simulink model "Reference_model_Control_Engineering_2022"  (R2022b)
settings: Solver=FixedStepDiscrete  StartTime=0.0  StopTime=inf  FixedStep=Ts  RelTol=1e-3  EnableMultiTasking=on
InitFcn:
  | Fs = 4000; Ts = 1/Fs; tsim = 29.9997;
settings Model: SimulationMode=external  ExtModeTrigDuration=2  Creator=Enzo  LastModifiedBy=vaish
settings SolverCC: AlgebraicLoopSolver=TrustRegion  PositivePriorityOrder=on
settings DataIOCC: SaveOutput=off  DSMLogging=off  SaveTime=off  ReturnWorkspaceOutputs=off
settings OptimizationCC: ReuseModelBlockBuffer=on  EnhancedBackFolding=on  PassReuseOutputArgsThreshold=0  MaxStackSize=64  OptimizeBlockOrder=speed  DifferentSizesBufferReuse=on  OptimizationCustomize=off
settings DebuggingCC: ParameterTunabilityLossMsg=error  UnconnectedInputMsg=warning  UnconnectedOutputMsg=warning  UnconnectedLineMsg=warning  ArithmeticOperatorsInVariantConditions=warning
settings HardwareCC: ProdBitPerPointer=32  ProdBitPerSizeT=32  ProdBitPerPtrDiffT=32  ProdLargestAtomicInteger=Long  ProdLargestAtomicFloat=Double  ProdWordSize=32  ProdLongLongMode=on  ProdHWDeviceType=ARM Compatible->ARM Cortex  UseEmbeddedCoderFeatures=off
settings ModelReferenceCC: EnableRefExpFcnMdlSchedulingChecks=on
settings SFSimCC: CustomCodeUndefinedFunction=UseInterfaceOnly
settings RTWCC: Description=Embedded Coder  SystemTargetFile=ert.tlc  HardwareBoard=Raspberry Pi  TLCOptions="-aInlineSetEventsForThisBaseRateFcn=TLC_FALSE -aSuppressMultiTaskScheduler=TLC_FALSE  -aRateBasedStepFcn=0"  TemplateMakefile=ert_default_tmf  PostCodeGenCommand="if (~verLessThan('matlab', '9.11')) codertarget.postCodeGenHookCommand(h);  SPERTE_postGenFunc(modelName, buildInfo); else; SPERTE_postGenFunc(h, buildInfo); end"  Toolchain=GNU GCC Embedded Linux  BuildConfiguration=Faster Runs
settings CodeAppCC: ForceParamTrailComments=on  OperatorAnnotations=on
settings ERTTargetCC: ERTCustomFileBanners=off  SupportContinuousTime=on  SupportNonInlinedSFcns=on  RemoveResetFunc=off  SupportVariableSizeSignals=on  ModelStepFunctionPrototypeControlCompliant=off  ExtMode=on  ExtModeMexArgs='sperte0.bwk.tue.nl' 0 17725  ERTSrcFileBannerTemplate=codertarget_code_template.cgt  ERTHdrFileBannerTemplate=codertarget_code_template.cgt  ERTDataSrcFileTemplate=codertarget_code_template.cgt  ERTDataHdrFileTemplate=codertarget_code_template.cgt
settings SettingsController: UseSoCProfilerForTargets=0

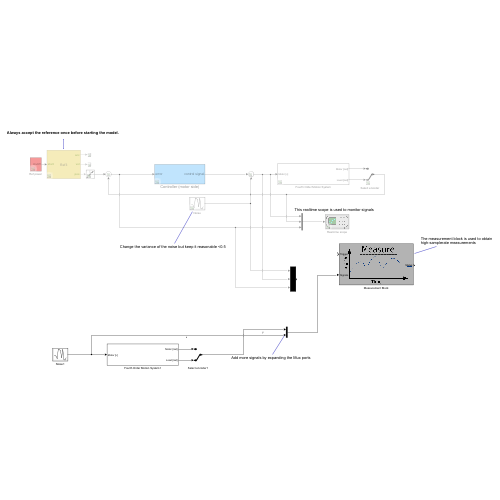
[thumbnail: Simulink's stored preview of the top-level diagram]
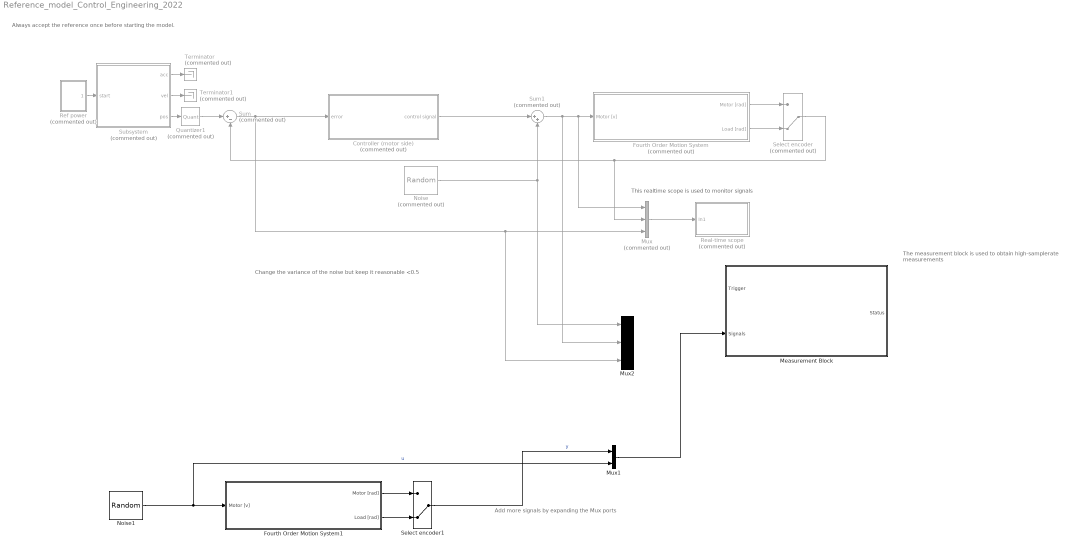
== system Reference_model_Control_Engineering_2022 ==
  note: Add more signals by expanding the Mux ports
  note: The measurement block is used to obtain high-samplerate measurements
  note: This realtime scope is used to monitor signals
  note: Always accept the reference once before starting the model.
  note: Change the variance of the noise but keep it reasonable <0.5
  Controller (motor side) : Subsystem  Commented=on
  Fourth Order Motion System : Subsystem  Commented=on
  Fourth Order Motion System1 : Subsystem
  Measurement Block : Subsystem  Description=|  Priority=-1  mask(SPERTE Lib){N_samples=480000, triggertype=2, trigger_command=0}
      | Perform on-demand measurements to file using this block.
      | 
      | It can be used in 2 ways:
      | 1) Set the mask triggertype parameter to manual and use the trigger input signal to trigger a measurement.
      | You can do this by providing a 0 to 1 transition.
      | Keep it low after you start/complete the measurement, or it will measure again.
      | A file is created with measurement_0,1,2... etc
      | 
      | 2) Keep the model running, and trigger a measurement from the commandline or Matlab script.
      | For example:
      | 
      | % How many samples to measure?
      | N_samples = Fs*5;
      | % Do the measurement
      | SPERTE_Perform_Measurement(N_samples);
      | % Get the latest file
      | file_list = SPERTE_Get_Latest_Measurement(p,1,'./data');
      | % How many signals did you record?
      | N_signals = 3;
      | % Convert the .bin to .mat and return the results
      | measurement = SPERTE_Bin_To_Mat(file_list,N_signals);
      mask prompts: N_samples "Number of samples"; trigger_command "Trigger command"
      mask help:
      | This block implements a measurement to file sink.
      | It can be used in two ways:
      | 1) Triggered from the simulink model
      | 2) Triggered from the command line
      mask Help:
      | Perform on-demand measurements to file using this block.
      | 
      | It can be used in 2 ways:
      | 1) Set the mask triggertype parameter to manual and use the trigger input signal to trigger a measurement.
      | You can do this by providing a 0 to 1 transition.
      | Keep it low after you start/complete the measurement, or it will measure again.
      | A file is created with measurement_0,1,2... etc
      | 
      | 2) Keep the model running, and trigger a measurement from the commandline or Matlab script.
      | For example:
      | 
      | % How many samples to measure?
      | N_samples = Fs*5;
      | % Do the measurement
      | SPERTE_Perform_Measurement(N_samples);
      | % Get the latest file
      | file_list = SPERTE_Get_Latest_Measurement(p,1,'./data');
      | % How many signals did you record?
      | N_signals = 3;
      | % Convert the .bin to .mat and return the results
      | measurement = SPERTE_Bin_To_Mat(file_list,N_signals);
      mask TypeOptions N_samples: SPERTE_measurement_samples/Value
      mask TypeOptions trigger_command: SPERTE_measurement_trigger_command/Value
      mask DialogControl BlockName Prompt: Sperte measurement block.
      mask DialogControl Desc Prompt: Can be used to trace signals to .bin file on the Raspberry Pi.  Can be triggered through signals in the simulink model or manually.
      mask DialogControl TriggerText Prompt: Manual (0), Command (1), Both (2)
      mask Display: ud = get_param(gcb,'UserData');image(ud.x);
  Mux : Mux  Commented=on  Inputs=3
  Mux1 : Mux  Inputs=2
  Mux2 : Mux  Inputs=3
  Noise : RandomNumber  Commented=on  SampleTime=Ts
  Noise1 : RandomNumber  SampleTime=Ts
  Quantizer1 : Quantizer  Commented=on  QuantizationInterval=(2*pi)/(500*4)
  Real-time scope : Subsystem  Priority=0  Commented=on  mask(Scope){Sample_Time=1/500}
      mask prompts: Sample_Time "Scope sample time"
      mask help:
      | Realtime Scope block allows one to view the signals while the model is running.
      | The signals are downsampled to a specified sample rate (in the mask parameter) to reduce communication overhead.
      settings: CopyFcn=set_param(gcb,'LinkStatus','None')  OpenFcn=open_system(strcat(get_param(gcb,'Parent'),'/',get_param(gcb,'Name'),'/Live_Scope'),'force');
      mask TypeOptions Sample_Time: Downsample/OutPortSampleTime
      mask DialogControl scopebutton Prompt: Open the live scope
      mask DialogControl scopebutton Callback: open_system(strcat(get_param(gcb,'Parent'),'/',get_param(gcb,'Name'),'/Live_Scope'));
      mask Display: ud = get_param(gcb,'UserData');image(ud.x);
  Ref power : Subsystem  Commented=on  mask(On/Off Switch){stat=Off}
      mask prompts: stat "Switch"
      mask TypeOptions stat: On | Off
  Select encoder : ManualSwitch  Commented=on  CurrentSetting=0
  Select encoder1 : ManualSwitch  CurrentSetting=0
  Subsystem : Subsystem  Commented=on  mask(Ref3){}
      settings: OpenFcn=global ref_part; cb_axes 1
      mask Display: disp('Ref3');
  Sum : Sum  Commented=on  Inputs=|+-
  Sum1 : Sum  Commented=on  Inputs=|++
  Terminator : Terminator  Commented=on
  Terminator1 : Terminator  Commented=on
  wires:
  Fourth Order Motion System/1(Motor [rad]) -> Select encoder/1
  Fourth Order Motion System/2(Load [rad]) -> Select encoder/2
  Select encoder/1 -> Mux/2, Sum/2
  Sum1/1 -> Mux2/2, Mux/1, Fourth Order Motion System/1(Motor [v])
  Controller (motor side)/1(control signal) -> Sum1/1
  Ref power/1(On/Off) -> Subsystem/1(start)
  Subsystem/3(pos) -> Quantizer1/1
  Mux/1 -> Real-time scope/1(In1)
  Noise/1 -> Mux2/1, Sum1/2
  Subsystem/1(acc) -> Terminator/1
  Subsystem/2(vel) -> Terminator1/1
  Noise1/1 -> Mux1/2, Fourth Order Motion System1/1(Motor [v])  "u"
  Fourth Order Motion System1/1(Motor [rad]) -> Select encoder1/1
  Select encoder1/1 -> Mux1/1  "y"
  Fourth Order Motion System1/2(Load [rad]) -> Select encoder1/2
  Sum/1 -> Mux2/3, Mux/3, Controller (motor side)/1(error)
  Quantizer1/1 -> Sum/1
  Mux1/1 -> Measurement Block/2(Signals)

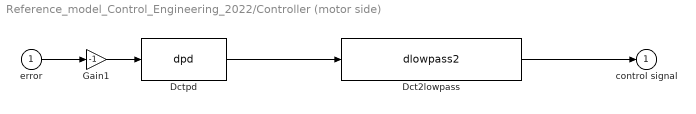
== system Reference_model_Control_Engineering_2022/Controller (motor side) ==
  error : Inport
  Dct2lowpass : S-Function  FunctionName=dlowpass2  Parameters=f_den, b_den, 0.001  SFunctionDeploymentMode=off  EnableBusSupport=off  mask(dctools){f_den=200, b_den=0.7}
      mask prompts: f_den "Pole [Hz]"; b_den "Damping pole [-]"
      mask help: This block implements a discrete time 2nd order lowpass filter.
      mask Display: disp('DCT 2nd order lowpass')
  Dctpd : S-Function  FunctionName=dpd  Parameters=kp, kv, 0.001  SFunctionDeploymentMode=off  EnableBusSupport=off  mask(dctools){kp=0.1, kv=0.001}
      mask help: This block implements a discrete time pd filter.
      mask Display: disp('DCT pd')
  Gain1 : Gain  Gain=-1  SaturateOnIntegerOverflow=on  OutDataTypeStr=Inherit: Same as input  ParamDataTypeStr=Inherit: Same as input
  control signal : Outport
  wires:
  Dct2lowpass/1 -> control signal/1
  Gain1/1 -> Dctpd/1
  error/1 -> Gain1/1
  Dctpd/1 -> Dct2lowpass/1

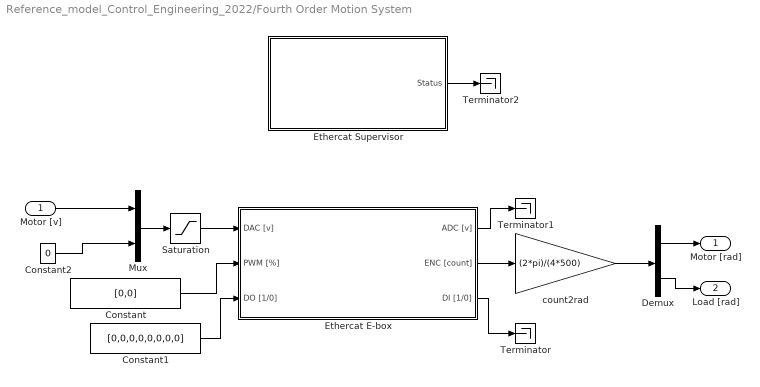
== system Reference_model_Control_Engineering_2022/Fourth Order Motion System ==
  Motor [v] : Inport
  Constant : Constant  Value=[0,0]
  Constant1 : Constant  Value=[0,0,0,0,0,0,0,0]
  Constant2 : Constant  Value=0
  Demux : Demux  Outputs=2
  Ethercat E-box : Subsystem  Priority=-2  mask(Sperte Lib){link_id=0}
      mask prompts: link_id "Link ID of the specific ebox"
      mask help:
      | This block implements a single E-box device.
      | Ensure that if you have multiple E-box devices that they each have an unique link_id.
      |
      | You MUST have an Ethercat Initialize block in your model to be able to use this block.
      mask Display: ud = get_param(gcb,'UserData');image(ud.x);
  Ethercat Supervisor : Subsystem  Description=Must be executed first, keep at -1 priority (highest)  Priority=-3  mask(Sperte Lib){portid=0, ectimeout=500}
      mask prompts: portid "Ethernet port number for the Ethercat protocol (default 0 = eth0)"; ectimeout "Timeout of the Ethercat protocol in microseconds."
      mask help:
      | This block initializes the Ethercat connection on the Raspberry Pi.
      |
      | This enables you to use multiple E-box devices by including multiple blocks of the "Ethercat E-box" type.
      mask Display: ud = get_param(gcb,'UserData');image(ud.x);
  Mux : Mux  Inputs=2
  Saturation : Saturate  UpperLimit=2.5  LowerLimit=-2.5
  Terminator : Terminator
  Terminator1 : Terminator
  Terminator2 : Terminator
  count2rad : Gain  Gain=(2*pi)/(4*500)
  Motor [rad] : Outport
  Load [rad] : Outport  Port=2
  wires:
  Ethercat E-box/1(ADC [v]) -> Terminator1/1
  Ethercat E-box/2(ENC [count]) -> count2rad/1
  Constant/1 -> Ethercat E-box/2(PWM [%])
  Mux/1 -> Saturation/1
  count2rad/1 -> Demux/1
  Motor [v]/1 -> Mux/1
  Constant2/1 -> Mux/2
  Demux/1 -> Motor [rad]/1
  Demux/2 -> Load [rad]/1
  Ethercat E-box/3(DI [1/0]) -> Terminator/1
  Constant1/1 -> Ethercat E-box/3(DO [1/0])
  Saturation/1 -> Ethercat E-box/1(DAC [v])
  Ethercat Supervisor/1(Status) -> Terminator2/1

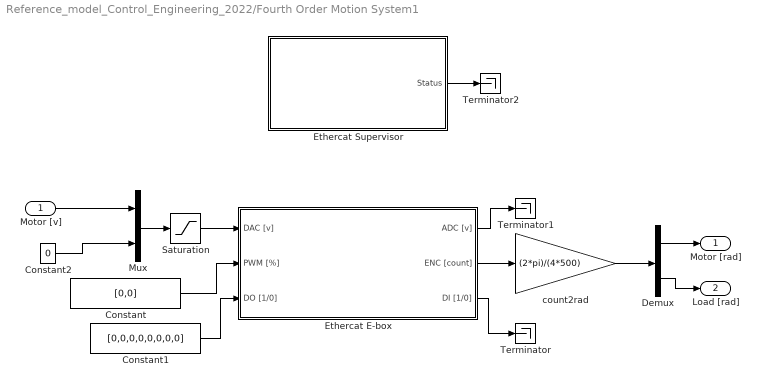
== system Reference_model_Control_Engineering_2022/Fourth Order Motion System1 ==
  Motor [v] : Inport
  Constant : Constant  Value=[0,0]
  Constant1 : Constant  Value=[0,0,0,0,0,0,0,0]
  Constant2 : Constant  Value=0
  Demux : Demux  Outputs=2
  Ethercat E-box : Subsystem  Priority=-2  mask(Sperte Lib){link_id=0}
      mask prompts: link_id "Link ID of the specific ebox"
      mask help:
      | This block implements a single E-box device.
      | Ensure that if you have multiple E-box devices that they each have an unique link_id.
      |
      | You MUST have an Ethercat Initialize block in your model to be able to use this block.
      mask Display: ud = get_param(gcb,'UserData');image(ud.x);
  Ethercat Supervisor : Subsystem  Description=Must be executed first, keep at -1 priority (highest)  Priority=-3  mask(Sperte Lib){portid=0, ectimeout=500}
      mask prompts: portid "Ethernet port number for the Ethercat protocol (default 0 = eth0)"; ectimeout "Timeout of the Ethercat protocol in microseconds."
      mask help:
      | This block initializes the Ethercat connection on the Raspberry Pi.
      |
      | This enables you to use multiple E-box devices by including multiple blocks of the "Ethercat E-box" type.
      mask Display: ud = get_param(gcb,'UserData');image(ud.x);
  Mux : Mux  Inputs=2
  Saturation : Saturate  UpperLimit=2.5  LowerLimit=-2.5
  Terminator : Terminator
  Terminator1 : Terminator
  Terminator2 : Terminator
  count2rad : Gain  Gain=(2*pi)/(4*500)
  Motor [rad] : Outport
  Load [rad] : Outport  Port=2
  wires:
  Ethercat Supervisor/1(Status) -> Terminator2/1
  Saturation/1 -> Ethercat E-box/1(DAC [v])
  Constant1/1 -> Ethercat E-box/3(DO [1/0])
  Ethercat E-box/3(DI [1/0]) -> Terminator/1
  Demux/2 -> Load [rad]/1
  Demux/1 -> Motor [rad]/1
  Constant2/1 -> Mux/2
  Motor [v]/1 -> Mux/1
  count2rad/1 -> Demux/1
  Mux/1 -> Saturation/1
  Constant/1 -> Ethercat E-box/2(PWM [%])
  Ethercat E-box/2(ENC [count]) -> count2rad/1
  Ethercat E-box/1(ADC [v]) -> Terminator1/1

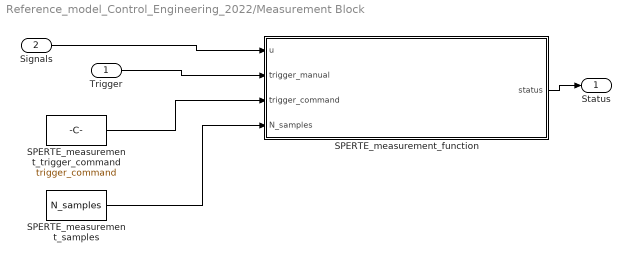
== system Reference_model_Control_Engineering_2022/Measurement Block ==
  Trigger : Inport
  Signals : Inport  Port=2
  SPERTE_measurement_function : MATLAB Function  TreatAsAtomicUnit=on
  SPERTE_measurement_samples : Constant  Value=N_samples  OutDataTypeStr=uint32
  SPERTE_measurement_trigger_command : Constant  Value=trigger_command  OutDataTypeStr=uint8
  Status : Outport
  wires:
  SPERTE_measurement_samples/1 -> SPERTE_measurement_function/4(N_samples)
  SPERTE_measurement_trigger_command/1 -> SPERTE_measurement_function/3(trigger_command)
  Signals/1 -> SPERTE_measurement_function/1(u)
  Trigger/1 -> SPERTE_measurement_function/2(trigger_manual)
  SPERTE_measurement_function/1(status) -> Status/1

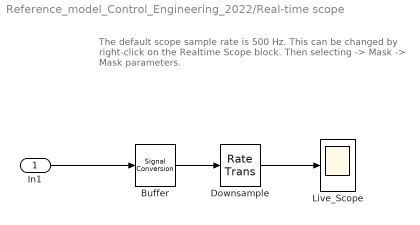
== system Reference_model_Control_Engineering_2022/Real-time scope ==
  note: The default scope sample rate is 500 Hz.
      | This can be changed by right-click on the Realtime Scope block.
      | Then selecting -> Mask -> Mask parameters.
  In1 : Inport
  Buffer : SignalConversion  OverrideOpt=off
  Downsample : RateTransition  OutPortSampleTime=Sample_Time
  Live_Scope : Scope
  wires:
  In1/1 -> Buffer/1
  Downsample/1 -> Live_Scope/1
  Buffer/1 -> Downsample/1

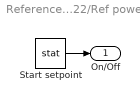
== system Reference_model_Control_Engineering_2022/Ref power ==
  Start setpoint : Constant  Value=stat
  On/Off : Outport
  wires:
  Start setpoint/1 -> On/Off/1

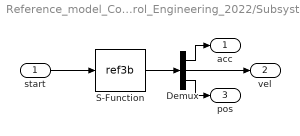
== system Reference_model_Control_Engineering_2022/Subsystem ==
  start : Inport
  Demux : Demux  Outputs=3
      settings: DisplayOption=none
  S-Function : S-Function  FunctionName=ref3b  Parameters=ref_part  SFunctionDeploymentMode=off  EnableBusSupport=off
      settings: OpenFcn=global ref_part; r3g_main
  acc : Outport
  vel : Outport  Port=2
  pos : Outport  Port=3
  wires:
  S-Function/1 -> Demux/1
  Demux/1 -> acc/1
  Demux/2 -> vel/1
  Demux/3 -> pos/1
  start/1 -> S-Function/1

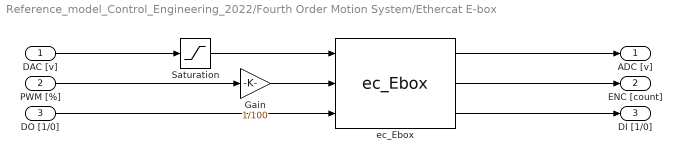
== system Reference_model_Control_Engineering_2022/Fourth Order Motion System/Ethercat E-box ==
  DAC [v] : Inport
  PWM [%] : Inport  Port=2
  DO [1/0] : Inport  Port=3
  Gain : Gain  Gain=1/100
  Saturation : Saturate  UpperLimit=10  LowerLimit=-10
  ec_Ebox : S-Function  FunctionName=ec_Ebox  Parameters=link_id  SFunctionDeploymentMode=off  EnableBusSupport=off  mask{link_id=link_id}
      mask prompts: link_id "link_id >= 0"
      mask Display:
      | port_label('output',1,'ADC')
      | port_label('output',2,'ENC')
      | port_label('output',3,'DI')
      | port_label('input',1,'DAC')
      | port_label('input',2,'PWM')
      | port_label('input',3,'DO')
  ADC [v] : Outport
  ENC [count] : Outport  Port=2
  DI [1/0] : Outport  Port=3
  wires:
  Gain/1 -> ec_Ebox/2
  Saturation/1 -> ec_Ebox/1
  ec_Ebox/3 -> DI [1/0]/1
  ec_Ebox/1 -> ADC [v]/1
  ec_Ebox/2 -> ENC [count]/1
  DAC [v]/1 -> Saturation/1
  DO [1/0]/1 -> ec_Ebox/3
  PWM [%]/1 -> Gain/1

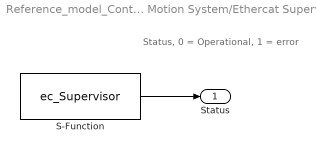
== system Reference_model_Control_Engineering_2022/Fourth Order Motion System/Ethercat Supervisor ==
  note: Status, 0 = Operational, 1 = error
  S-Function : S-Function  FunctionName=ec_Supervisor  Parameters=portid,ectimeout  SFunctionDeploymentMode=off  EnableBusSupport=off
  Status : Outport
  wires:
  S-Function/1 -> Status/1

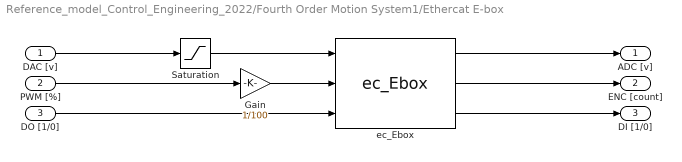
== system Reference_model_Control_Engineering_2022/Fourth Order Motion System1/Ethercat E-box ==
  DAC [v] : Inport
  PWM [%] : Inport  Port=2
  DO [1/0] : Inport  Port=3
  Gain : Gain  Gain=1/100
  Saturation : Saturate  UpperLimit=10  LowerLimit=-10
  ec_Ebox : S-Function  FunctionName=ec_Ebox  Parameters=link_id  SFunctionDeploymentMode=off  EnableBusSupport=off  mask{link_id=link_id}
      mask prompts: link_id "link_id >= 0"
      mask Display:
      | port_label('output',1,'ADC')
      | port_label('output',2,'ENC')
      | port_label('output',3,'DI')
      | port_label('input',1,'DAC')
      | port_label('input',2,'PWM')
      | port_label('input',3,'DO')
  ADC [v] : Outport
  ENC [count] : Outport  Port=2
  DI [1/0] : Outport  Port=3
  wires:
  PWM [%]/1 -> Gain/1
  DO [1/0]/1 -> ec_Ebox/3
  DAC [v]/1 -> Saturation/1
  ec_Ebox/2 -> ENC [count]/1
  ec_Ebox/1 -> ADC [v]/1
  ec_Ebox/3 -> DI [1/0]/1
  Saturation/1 -> ec_Ebox/1
  Gain/1 -> ec_Ebox/2

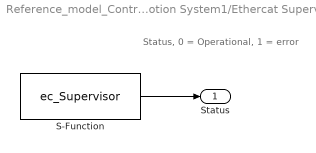
== system Reference_model_Control_Engineering_2022/Fourth Order Motion System1/Ethercat Supervisor ==
  note: Status, 0 = Operational, 1 = error
  S-Function : S-Function  FunctionName=ec_Supervisor  Parameters=portid,ectimeout  SFunctionDeploymentMode=off  EnableBusSupport=off
  Status : Outport
  wires:
  S-Function/1 -> Status/1

== matlab function Reference_model_Control_Engineering_2022/Measurement Block/SPERTE_measurement_function ==
  data: u input double; status output uint8 size=[1]; trigger_manual input uint8 size=[1]; trigger_command input uint8 size=[1]; triggertype parameter uint8 size=[1]; N_samples input uint32 size=1
function status = perform_measurement(u, trigger_manual, trigger_command, triggertype, N_samples)

%% Persistent variables
persistent fileID NF busy NS

% Init parameters
if isempty(NF)
    NF = int16(0);
end
if isempty(NS)
    NS = uint32(0);
end
if isempty(fileID)
    fileID = 0;
end
if isempty(busy)
    busy = uint8(0);
end

%% Check the triggers
if ( (triggertype == 0 && trigger_manual == 1) || (triggertype == 1 && trigger_command == 1) || (triggertype == 2 && (trigger_command == 1 || trigger_manual == 1) ) )
    if busy == 1
        % We are already busy, nothing to do
    else
        % We should start a new one
        fileID = fopen(sprintf('measurement_%d.bin',NF),'w');  
        NF = NF + 1;
        busy = uint8(1);
        NS = uint32(0);
    end
end

% We have started a measurement
if busy == 1
    if NS < N_samples 
        % Here we write the sample, in single precision float
        fwrite(fileID,u,'single');
        NS = NS + uint32(1);
    else
       % We have N samples already, we are done
       fclose(fileID);
       busy = uint8(0);
       NS = uint32(0);
    end
      
end
    % Output state
    status = uint8(busy);
end
